simulink model "mat_double"  (R2020b)
settings: Solver=VariableStepAuto  StartTime=0.0  StopTime=10.0  RelTol=1e-3
values from neighbouring files (symbols this model uses):
  d1 = 0.5    [simu.m]    (also in simu_J1fix.m)
  d2 = 0.5    [simu.m]    (also in simu_J1fix.m)
  is_tm1 = 1    [simu.m]    (also in simu_J1fix.m)
  is_tm2 = 1    [simu.m]    (also in simu_J1fix.m)
  J1 = 1    [simu.m]    (also in simu_J1fix.m)
  J2 = 1    [simu.m]    (also in simu_J1fix.m = 0.8)
  k1 = 100    [simu.m]    (also in simu_J1fix.m)
  k2 = 100    [simu.m]    (also in simu_J1fix.m = 80)
undefined symbols (not defined in the file or in its folder): X, Y, Z
libraries: sm_lib x25, nesl_utility x17, fl_lib x6
settings Model: Creator=BearHsia  LastModifiedBy=BearHsia
settings ExplorerConfigSet: InternalSimMechanicsExplorerSettings="<ExplorerConfiguration><canonicalview>aerospace</canonicalview><AnimationSetting><BasePlaybackSpeed>1.0</BasePlaybackSpeed><PlaybackSpeedFactor>1.0</PlaybackSpeedFactor></AnimationSetting><TilePanel><TileInfo><Tiles Columns=\"1\" Count=\"1\" Rows=\"1\"><Column Weight=\"1\"/><Row Weight=\"1\"/><Tile Height=\"1\" Width=\"1\" X=\"0\" Y=\"0\"/></Tiles></TileInfo><SceneInfo><SceneViewer><BGColor><R>0.60000002384185791</R><G>0.60000002384185791</G><B>0.60000002384185791</B></BGColor><Camera><DoPerspective>off</DoPerspective><Position><X>0.0536048974703797823</X><Y>-0.0148520376451683166</Y><Z>1.01248960387817566</Z></Position><Center><X>0.0543519392340099453</X><Y>0.0174866883236047335</Y><Z>0.0130129164405163693</Z></Center><Up><X>-0.00285720568225904682</X><Y>0.999472955665096308</Y><Z>0.0323364696552736336</Z></Up><ViewLimDist>1</ViewLimDist><YLim>0.224098919359438681</YLim><XLim>0.18381667559028339</XLim></Camera></SceneViewer></SceneInfo></TilePanel><MechEditorPanel><Cameras/><GfxPanelCameraMap/><VideoCreator><PlaybackSpeedRatio>1.0</PlaybackSpeedRatio><FrameRate>30</FrameRate><VideoFormat>Motion JPEG AVI</VideoFormat><FrameSize>auto</FrameSize></VideoCreator></MechEditorPanel></ExplorerConfiguration>"

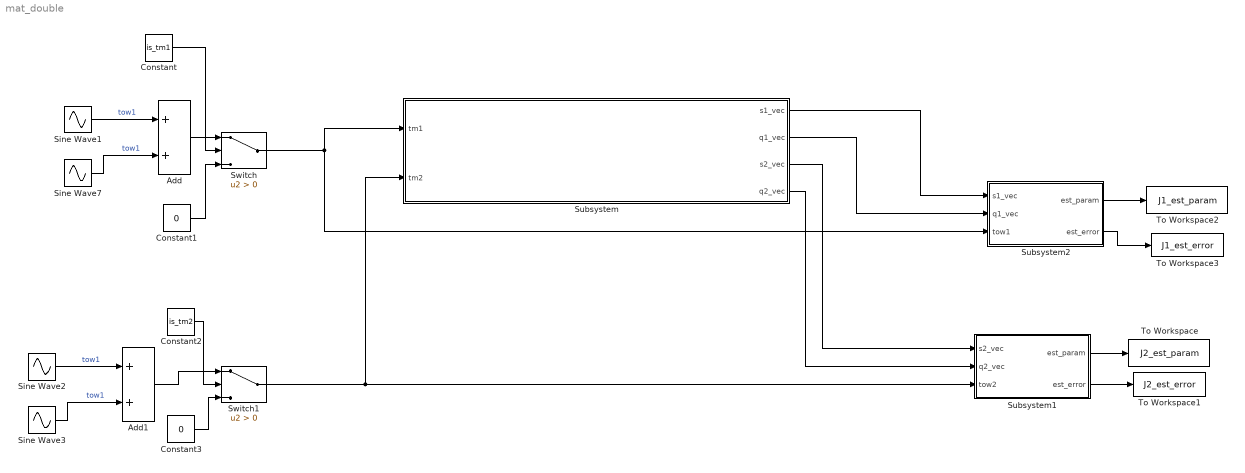
== system mat_double ==
  Add : Sum
  Add1 : Sum
  Constant : Constant  Value=is_tm1
  Constant1 : Constant  Value=0
  Constant2 : Constant  Value=is_tm2
  Constant3 : Constant  Value=0
  Sine Wave1 : Sin  Frequency=0.5  SampleTime=0
  Sine Wave2 : Sin  Amplitude=0.5  Frequency=0.5  SampleTime=0
  Sine Wave3 : Sin  Amplitude=0.25  Frequency=0.1  SampleTime=0
  Sine Wave7 : Sin  Amplitude=0.5  Frequency=0.1  SampleTime=0
  Subsystem : Subsystem
  Subsystem1 : Subsystem
  Subsystem2 : Subsystem
  Switch : Switch  Criteria=u2 > Threshold
  Switch1 : Switch  Criteria=u2 > Threshold
  To Workspace : ToWorkspace  VariableName=J2_est_param  SaveFormat=Timeseries  SampleTime=-1
  To Workspace1 : ToWorkspace  VariableName=J2_est_error  SaveFormat=Timeseries  SampleTime=-1
  To Workspace2 : ToWorkspace  VariableName=J1_est_param  SaveFormat=Timeseries  SampleTime=-1
  To Workspace3 : ToWorkspace  VariableName=J1_est_error  SaveFormat=Timeseries  SampleTime=-1
  wires:
  Constant1/1 -> Switch/3
  Constant/1 -> Switch/2
  Add/1 -> Switch/1
  Sine Wave7/1 -> Add/2  "tow1"
  Sine Wave1/1 -> Add/1  "tow1"
  Switch/1 -> Subsystem2/3(tow1), Subsystem/1(tm1)
  Subsystem2/2(est_error) -> To Workspace3/1
  Subsystem2/1(est_param) -> To Workspace2/1
  Subsystem/1(s1_vec) -> Subsystem2/1(s1_vec)
  Subsystem/2(q1_vec) -> Subsystem2/2(q1_vec)
  Add1/1 -> Switch1/1
  Constant2/1 -> Switch1/2
  Constant3/1 -> Switch1/3
  Sine Wave2/1 -> Add1/1  "tow1"
  Sine Wave3/1 -> Add1/2  "tow1"
  Switch1/1 -> Subsystem/2(tm2), Subsystem1/3(tow2)
  Subsystem1/1(est_param) -> To Workspace/1
  Subsystem1/2(est_error) -> To Workspace1/1
  Subsystem/3(s2_vec) -> Subsystem1/1(s2_vec)
  Subsystem/4(q2_vec) -> Subsystem1/2(q2_vec)

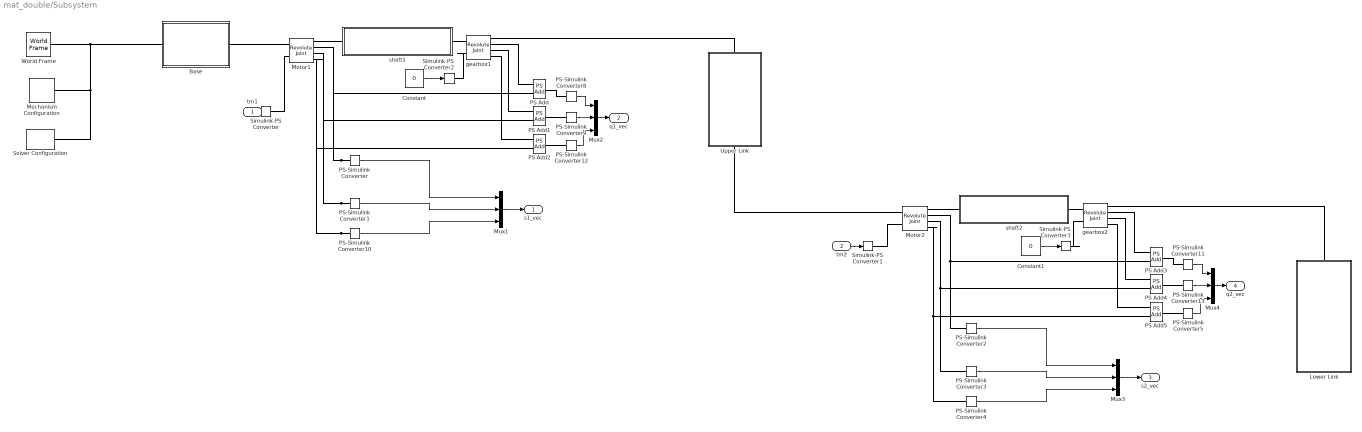
== system mat_double/Subsystem ==
  tm1 : Inport
  tm2 : Inport  Port=2
  Base : Subsystem  mask(Double Pendulum Base){R=6, T=0.5, rp=0.5, clr=[0.5 0.5 0.5], img_file=sm_dpen_base.png}
      mask prompts: R "Base radius (cm):"; T "Base thickness (cm):"; rp "Peg radius (cm):"; clr "Base color:"; img_file "Image file:"
      mask help: Base body of the double pendulum mechanism.
      mask Display: image(imread(img_file))
  Constant : Constant  Value=0
  Constant1 : Constant  Value=0
  Lower Link : Subsystem  mask(Lower Link){Ro=1200, L=20, W=2, T=0.5, r=0.5, clr=[1.0 0.2 0.2], img_file=sm_dpen_lower_link.png}
      mask prompts: Ro "Link density (kg/m^3):"; L "Link length (cm):"; W "Link width (cm):"; T "Link thickness (cm):"; r "Peg/Hole radius (cm):"; clr "Link color:"; img_file "Link image file:"
      mask help: Lower link of the pendulum mechanism.
      mask init:
      | % Main link cross-section
      | top_xsec = [L/2 W/2; -L/2 W/2];
      | theta = (90:-1:-90)*pi/180;
      | semi_hole_xsec = [-L/2+r*cos(theta') r*sin(theta')];
      | bottom_xsec = [-L/2 -W/2; L/2 -W/2];
      | theta = (-89:1:89)*pi/180;
      | right_end_xsec = [L/2+(W/2)*cos(theta') (W/2)*sin(theta')];
      | link_x_section = [ top_xsec; semi_hole_xsec; bottom_xsec; right_end_xsec];
      | 
      | % Left end cap cross-section
      | theta = (90:1:270)*pi/180;
      | outer_xsec = [(W/2)*cos(theta') (W/2)*sin(theta')];
      | theta = (270:-1:90)*pi/180;
      | inner_xsec = [r*cos(theta') r*sin(theta')];
      | left_end_x_section = [outer_xsec; inner_xsec];
      mask Display: image(imread(img_file));
  Mechanism Configuration : sm_lib/Utilities/Mechanism Configuration  UniformGravity=Constant  GravityVector=[0 -9.81 0]  GravityVectorUnits=m/s^2  GravityUnits=m/s^2  LinearizationDelta=0.001  JointModeTransitionNonlinearIterations=2
      settings: SourceProductName=Multibody
  Motor1 : sm_lib/Joints/Revolute Joint  JointMode=Normal  SenseConstraintForce=off  SenseConstraintForceX=off  SenseConstraintForceY=off  SenseConstraintForceZ=off  SenseConstraintTorque=off  SenseConstraintTorqueX=off  SenseConstraintTorqueY=off  SenseConstraintTorqueZ=off  SenseTotalForce=off  SenseTotalForceX=off  SenseTotalForceY=off  SenseTotalForceZ=off  SenseTotalTorque=off  SenseTotalTorqueX=off  SenseTotalTorqueY=off  SenseTotalTorqueZ=off  CompositeWrenchDir=FollowerOnBase  CompositeWrenchFrame=BaseFrame  EquilibriumPosition=0  EquilibriumPositionUnits=rad  SpringStiffness=0  SpringStiffnessUnits=N*m/rad  DampingCoefficient=0  DampingCoefficientUnits=N*m/(rad/s)  TorqueActuationMode=InputTorque  MotionActuationMode=ComputedMotion  SensePosition=on  SenseVelocity=on  SenseAcceleration=on  SenseTorqueForce=off  SenseLowerLimitTorqueForce=off  SenseUpperLimitTorqueForce=off  LowerLimitSpecify=off  LowerLimitBound=-90  LowerLimitBoundUnits=deg  LowerLimitStiffness=1e4  LowerLimitStiffnessUnits=N*m/deg  LowerLimitDamping=10  LowerLimitDampingUnits=N*m/(deg/s)  LowerLimitTransitionRegionWidth=0.1  LowerLimitTransitionRegionWidthUnits=deg  UpperLimitSpecify=off  UpperLimitBound=90  UpperLimitBoundUnits=deg  UpperLimitStiffness=1e4  UpperLimitStiffnessUnits=N*m/deg  UpperLimitDamping=10  UpperLimitDampingUnits=N*m/(deg/s)  UpperLimitTransitionRegionWidth=0.1  UpperLimitTransitionRegionWidthUnits=deg  PositionTargetSpecify=on  PositionTargetPriority=High  PositionTargetValue=0  PositionTargetValueUnits=rad  VelocityTargetSpecify=off  VelocityTargetPriority=High  VelocityTargetValue=0  VelocityTargetValueUnits=deg/s
  Motor2 : sm_lib/Joints/Revolute Joint  JointMode=Normal  SenseConstraintForce=off  SenseConstraintForceX=off  SenseConstraintForceY=off  SenseConstraintForceZ=off  SenseConstraintTorque=off  SenseConstraintTorqueX=off  SenseConstraintTorqueY=off  SenseConstraintTorqueZ=off  SenseTotalForce=off  SenseTotalForceX=off  SenseTotalForceY=off  SenseTotalForceZ=off  SenseTotalTorque=off  SenseTotalTorqueX=off  SenseTotalTorqueY=off  SenseTotalTorqueZ=off  CompositeWrenchDir=FollowerOnBase  CompositeWrenchFrame=BaseFrame  EquilibriumPosition=0  EquilibriumPositionUnits=rad  SpringStiffness=0  SpringStiffnessUnits=N*m/rad  DampingCoefficient=0  DampingCoefficientUnits=N*m/(rad/s)  TorqueActuationMode=InputTorque  MotionActuationMode=ComputedMotion  SensePosition=on  SenseVelocity=on  SenseAcceleration=on  SenseTorqueForce=off  SenseLowerLimitTorqueForce=off  SenseUpperLimitTorqueForce=off  LowerLimitSpecify=off  LowerLimitBound=-90  LowerLimitBoundUnits=deg  LowerLimitStiffness=1e4  LowerLimitStiffnessUnits=N*m/deg  LowerLimitDamping=10  LowerLimitDampingUnits=N*m/(deg/s)  LowerLimitTransitionRegionWidth=0.1  LowerLimitTransitionRegionWidthUnits=deg  UpperLimitSpecify=off  UpperLimitBound=90  UpperLimitBoundUnits=deg  UpperLimitStiffness=1e4  UpperLimitStiffnessUnits=N*m/deg  UpperLimitDamping=10  UpperLimitDampingUnits=N*m/(deg/s)  UpperLimitTransitionRegionWidth=0.1  UpperLimitTransitionRegionWidthUnits=deg  PositionTargetSpecify=on  PositionTargetPriority=High  PositionTargetValue=0  PositionTargetValueUnits=rad  VelocityTargetSpecify=off  VelocityTargetPriority=High  VelocityTargetValue=0  VelocityTargetValueUnits=deg/s
  Mux{1..4} (4 alike) : Mux  Inputs=3
  PS Add{,1..5} (6 alike) : fl_lib/Physical Signals/Functions/PS Add
  PS-Simulink Converter{,1..5,8..13} (12 alike) : nesl_utility/PS-Simulink Converter  PhysicalDomain=network_engine_domain  SubClassName=ps_output  LeftPortType=input  RightPortType=output  PseudoPeriodic=off  Frequencies=[]  Unit=inherit  AffineConversion=off
  Simulink-PS Converter{,1..3} (4 alike) : nesl_utility/Simulink-PS Converter  PhysicalDomain=network_engine_domain  SubClassName=ps_input  LeftPortType=input  RightPortType=output  PseudoPeriodic=off  Frequencies=[]  NoiseDistribution=none  NoiseParameters=[]  Unit=1  AffineConversion=off  FilteringAndDerivatives=provide  SimscapeFilterOrder=1  InputFilterTimeConstant=0.001  UdotUserProvided=0
  Solver Configuration : nesl_utility/Solver Configuration  PhysicalDomain=network_engine_domain  SubClassName=solver  LeftPortType=input  RightPortType=generic  Tones=[]  Harmonics=[]  SimulateNoise=off  Profile=off  UseLocalSampling=off  EnableSwitchedLinearOptims=on  FrequencyDomain=off  UseCCode=off  RelTol=0.001  AbsTol=1e-06  MinStep=1e-09  ToWorkspace=off  RevertToSquareIcSolve=off  NumHomotopyIterations=100  PhasorMode=off  PhasorModeNumHarmonics=1  DoDC=off  ResidualTolerance=1e-9  UseLocalSolver=off  LocalSolverChoice=NE_BACKWARD_EULER_ADVANCER  LocalSolverSampleTime=.001  DoFixedCost=off  MaxNonlinIter=3  MaxModeIter=2  ComputeImpulses=off  ImpulseIterations=2  LinearAlgebra=Sparse  EquationFormulation=NE_TIME_EF  DelaysMemoryBudget=1024  AutomaticFiltering=on  FilteringTimeConstant=0.001  PartitionStorageMethod=AS_NEEDED  PartitionMemoryBudget=1024  PartitionMethod=FAST
      settings: SourceProductName=Utilities
  Upper Link : Subsystem  mask(Upper Link){Ro=1000, L=14, W=2, T=0.5, r=0.5, clr=[0.0 0.6 0.8], img_file=sm_dpen_upper_link.png}
      mask prompts: Ro "Link density (kg/m^3):"; L "Link length (cm):"; W "Link width (cm):"; T "Link thickness (cm):"; r "Peg/Hole radius (cm):"; clr "Link color:"; img_file "Link image file:"
      mask help: Upper link of the double pendulum mechanism
      mask init: same as mat_double/Subsystem/Lower Link
      mask Display: image(imread(img_file));
  World Frame : sm_lib/Frames and Transforms/World Frame
      settings: SourceProductName=Multibody
  gearbox1 : sm_lib/Joints/Revolute Joint  JointMode=Normal  SenseConstraintForce=off  SenseConstraintForceX=off  SenseConstraintForceY=off  SenseConstraintForceZ=off  SenseConstraintTorque=off  SenseConstraintTorqueX=off  SenseConstraintTorqueY=off  SenseConstraintTorqueZ=off  SenseTotalForce=off  SenseTotalForceX=off  SenseTotalForceY=off  SenseTotalForceZ=off  SenseTotalTorque=off  SenseTotalTorqueX=off  SenseTotalTorqueY=off  SenseTotalTorqueZ=off  CompositeWrenchDir=FollowerOnBase  CompositeWrenchFrame=BaseFrame  EquilibriumPosition=0  EquilibriumPositionUnits=rad  SpringStiffness=k1  SpringStiffnessUnits=N*m/rad  DampingCoefficient=d1  DampingCoefficientUnits=N*m/(rad/s)  TorqueActuationMode=InputTorque  MotionActuationMode=ComputedMotion  SensePosition=on  SenseVelocity=on  SenseAcceleration=on  SenseTorqueForce=off  SenseLowerLimitTorqueForce=off  SenseUpperLimitTorqueForce=off  LowerLimitSpecify=off  LowerLimitBound=-90  LowerLimitBoundUnits=deg  LowerLimitStiffness=1e4  LowerLimitStiffnessUnits=N*m/deg  LowerLimitDamping=10  LowerLimitDampingUnits=N*m/(deg/s)  LowerLimitTransitionRegionWidth=0.1  LowerLimitTransitionRegionWidthUnits=deg  UpperLimitSpecify=off  UpperLimitBound=90  UpperLimitBoundUnits=deg  UpperLimitStiffness=1e4  UpperLimitStiffnessUnits=N*m/deg  UpperLimitDamping=10  UpperLimitDampingUnits=N*m/(deg/s)  UpperLimitTransitionRegionWidth=0.1  UpperLimitTransitionRegionWidthUnits=deg  PositionTargetSpecify=on  PositionTargetPriority=High  PositionTargetValue=0  PositionTargetValueUnits=rad  VelocityTargetSpecify=off  VelocityTargetPriority=High  VelocityTargetValue=0  VelocityTargetValueUnits=deg/s
  gearbox2 : sm_lib/Joints/Revolute Joint  JointMode=Normal  SenseConstraintForce=off  SenseConstraintForceX=off  SenseConstraintForceY=off  SenseConstraintForceZ=off  SenseConstraintTorque=off  SenseConstraintTorqueX=off  SenseConstraintTorqueY=off  SenseConstraintTorqueZ=off  SenseTotalForce=off  SenseTotalForceX=off  SenseTotalForceY=off  SenseTotalForceZ=off  SenseTotalTorque=off  SenseTotalTorqueX=off  SenseTotalTorqueY=off  SenseTotalTorqueZ=off  CompositeWrenchDir=FollowerOnBase  CompositeWrenchFrame=BaseFrame  EquilibriumPosition=0  EquilibriumPositionUnits=rad  SpringStiffness=k2  SpringStiffnessUnits=N*m/rad  DampingCoefficient=d2  DampingCoefficientUnits=N*m/(rad/s)  TorqueActuationMode=InputTorque  MotionActuationMode=ComputedMotion  SensePosition=on  SenseVelocity=on  SenseAcceleration=on  SenseTorqueForce=off  SenseLowerLimitTorqueForce=off  SenseUpperLimitTorqueForce=off  LowerLimitSpecify=off  LowerLimitBound=-90  LowerLimitBoundUnits=deg  LowerLimitStiffness=1e4  LowerLimitStiffnessUnits=N*m/deg  LowerLimitDamping=10  LowerLimitDampingUnits=N*m/(deg/s)  LowerLimitTransitionRegionWidth=0.1  LowerLimitTransitionRegionWidthUnits=deg  UpperLimitSpecify=off  UpperLimitBound=90  UpperLimitBoundUnits=deg  UpperLimitStiffness=1e4  UpperLimitStiffnessUnits=N*m/deg  UpperLimitDamping=10  UpperLimitDampingUnits=N*m/(deg/s)  UpperLimitTransitionRegionWidth=0.1  UpperLimitTransitionRegionWidthUnits=deg  PositionTargetSpecify=on  PositionTargetPriority=High  PositionTargetValue=0  PositionTargetValueUnits=rad  VelocityTargetSpecify=off  VelocityTargetPriority=High  VelocityTargetValue=0  VelocityTargetValueUnits=deg/s
  shaft1 : Subsystem  mask{rgb=[0 1 0], Ixx=0, Iyy=0, Izz=J1, M=0.1, L=0.2, W=0.004, H=0.004}
      mask prompts: rgb "Color [R G B]"
  shaft2 : Subsystem  mask{rgb=[0 1 0], Ixx=0, Iyy=0, Izz=J2, M=0.1, L=0.2, W=0.004, H=0.004}
      mask prompts: rgb "Color [R G B]"
  s1_vec : Outport
  q1_vec : Outport  Port=2
  s2_vec : Outport  Port=3
  q2_vec : Outport  Port=4
  wires:
  PS-Simulink Converter/1 -> Mux1/1
  PS-Simulink Converter8/1 -> Mux2/1
  PS-Simulink Converter9/1 -> Mux2/2
  Constant/1 -> Simulink-PS Converter2/1
  Mux2/1 -> q1_vec/1
  PS-Simulink Converter1/1 -> Mux1/2
  PS-Simulink Converter10/1 -> Mux1/3
  tm1/1 -> Simulink-PS Converter/1
  Mux1/1 -> s1_vec/1
  PS-Simulink Converter12/1 -> Mux2/3
  Constant1/1 -> Simulink-PS Converter3/1
  PS-Simulink Converter11/1 -> Mux4/1
  PS-Simulink Converter4/1 -> Mux3/3
  PS-Simulink Converter3/1 -> Mux3/2
  Mux3/1 -> s2_vec/1
  Mux4/1 -> q2_vec/1
  PS-Simulink Converter13/1 -> Mux4/2
  PS-Simulink Converter2/1 -> Mux3/1
  PS-Simulink Converter5/1 -> Mux4/3
  tm2/1 -> Simulink-PS Converter1/1
  connections:
  Base/RConn1 -- Motor1/LConn1
  Mechanism Configuration/RConn1 -- Solver Configuration/RConn1 -- Base/LConn1 -- World Frame/RConn1
  Motor2/LConn1 -- Upper Link/RConn1
  gearbox1/RConn1 -- Upper Link/LConn1
  PS-Simulink Converter/LConn1 -- Motor1/RConn2 -- PS Add/LConn2
  PS-Simulink Converter1/LConn1 -- Motor1/RConn3 -- PS Add1/LConn2
  PS-Simulink Converter10/LConn1 -- Motor1/RConn4 -- PS Add2/LConn2
  PS Add1/RConn1 -- PS-Simulink Converter9/LConn1
  shaft1/LConn1 -- Motor1/RConn1
  gearbox1/RConn2 -- PS Add/LConn1
  gearbox1/RConn4 -- PS Add2/LConn1
  Simulink-PS Converter/RConn1 -- Motor1/LConn2
  shaft1/RConn1 -- gearbox1/LConn1
  gearbox1/LConn2 -- Simulink-PS Converter2/RConn1
  PS Add/RConn1 -- PS-Simulink Converter8/LConn1
  gearbox1/RConn3 -- PS Add1/LConn1
  PS-Simulink Converter12/LConn1 -- PS Add2/RConn1
  PS Add4/LConn2 -- PS-Simulink Converter3/LConn1 -- Motor2/RConn3
  PS Add5/LConn2 -- PS-Simulink Converter4/LConn1 -- Motor2/RConn4
  PS Add3/LConn2 -- PS-Simulink Converter2/LConn1 -- Motor2/RConn2
  Simulink-PS Converter1/RConn1 -- Motor2/LConn2
  Simulink-PS Converter3/RConn1 -- gearbox2/LConn2
  shaft2/RConn1 -- gearbox2/LConn1
  shaft2/LConn1 -- Motor2/RConn1
  gearbox2/RConn4 -- PS Add5/LConn1
  gearbox2/RConn2 -- PS Add3/LConn1
  PS-Simulink Converter5/LConn1 -- PS Add5/RConn1
  gearbox2/RConn3 -- PS Add4/LConn1
  PS Add3/RConn1 -- PS-Simulink Converter11/LConn1
  Lower Link/LConn1 -- gearbox2/RConn1
  PS Add4/RConn1 -- PS-Simulink Converter13/LConn1

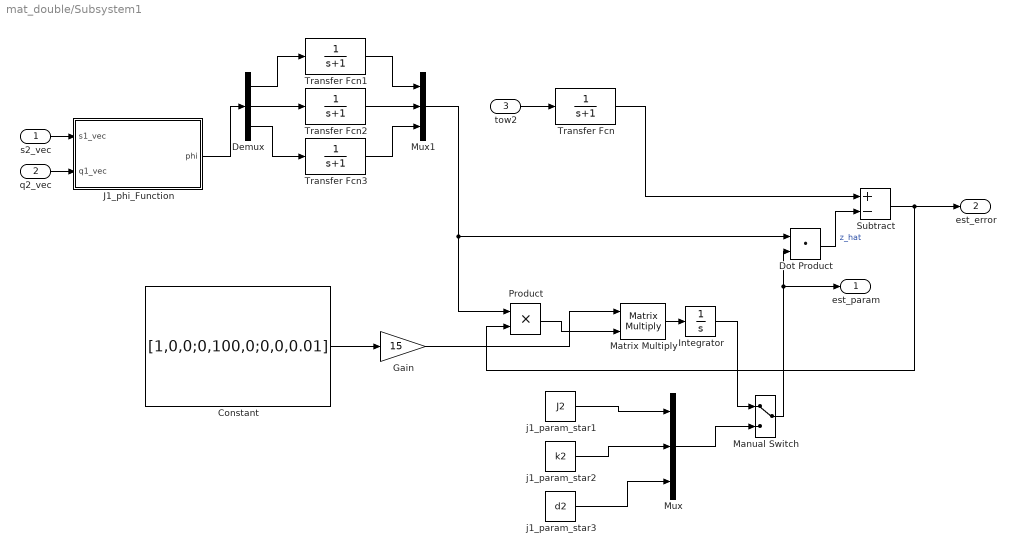
== system mat_double/Subsystem1 ==
  s2_vec : Inport
  q2_vec : Inport  Port=2
  tow2 : Inport  Port=3
  Constant : Constant  Value=[1,0,0;0,100,0;0,0,0.01]
  Demux : Demux  Outputs=3
  Dot Product : DotProduct  InputSameDT=on  OutDataTypeStr=Inherit: Inherit via internal rule
  Gain : Gain  Gain=15
  Integrator : Integrator  InitialCondition=[0.0001;0.0001;0.0001]
  J1_phi_Function : MATLAB Function  TreatAsAtomicUnit=on
  Manual Switch : ManualSwitch
  Matrix Multiply : Product  Multiplication=Matrix(*)
  Mux : Mux  Inputs=3
  Mux1 : Mux  Inputs=3
  Product : Product
  Subtract : Sum  Inputs=+-
  Transfer Fcn{,1..3} (4 alike) : TransferFcn  Denominator=[1 1]
  j1_param_star1 : Constant  Value=J2
  j1_param_star2 : Constant  Value=k2
  j1_param_star3 : Constant  Value=d2
  est_param : Outport
  est_error : Outport  Port=2
  wires:
  q2_vec/1 -> J1_phi_Function/2(q1_vec)
  s2_vec/1 -> J1_phi_Function/1(s1_vec)
  Integrator/1 -> Manual Switch/1
  tow2/1 -> Transfer Fcn/1
  Dot Product/1 -> Subtract/2  "z_hat"
  Matrix Multiply/1 -> Integrator/1
  Subtract/1 -> est_error/1, Product/2
  j1_param_star1/1 -> Mux/1
  j1_param_star2/1 -> Mux/2
  j1_param_star3/1 -> Mux/3
  Mux/1 -> Manual Switch/2
  Product/1 -> Matrix Multiply/2
  Constant/1 -> Gain/1
  Gain/1 -> Matrix Multiply/1
  J1_phi_Function/1(phi) -> Demux/1
  Manual Switch/1 -> est_param/1, Dot Product/2
  Transfer Fcn/1 -> Subtract/1
  Transfer Fcn1/1 -> Mux1/1
  Transfer Fcn2/1 -> Mux1/2
  Transfer Fcn3/1 -> Mux1/3
  Demux/3 -> Transfer Fcn3/1
  Demux/2 -> Transfer Fcn2/1
  Demux/1 -> Transfer Fcn1/1
  Mux1/1 -> Product/1, Dot Product/1

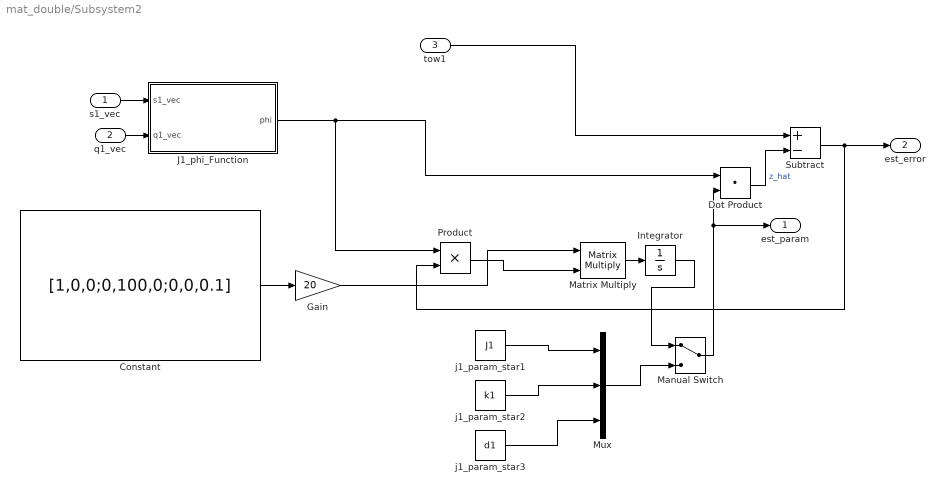
== system mat_double/Subsystem2 ==
  s1_vec : Inport
  q1_vec : Inport  Port=2
  tow1 : Inport  Port=3
  Constant : Constant  Value=[1,0,0;0,100,0;0,0,0.1]
  Dot Product : DotProduct  InputSameDT=on  OutDataTypeStr=Inherit: Inherit via internal rule
  Gain : Gain  Gain=20
  Integrator : Integrator  InitialCondition=[0;0;0]
  J1_phi_Function : MATLAB Function  TreatAsAtomicUnit=on
  Manual Switch : ManualSwitch
  Matrix Multiply : Product  Multiplication=Matrix(*)
  Mux : Mux  Inputs=3
  Product : Product
  Subtract : Sum  Inputs=+-
  j1_param_star1 : Constant  Value=J1
  j1_param_star2 : Constant  Value=k1
  j1_param_star3 : Constant  Value=d1
  est_param : Outport
  est_error : Outport  Port=2
  wires:
  q1_vec/1 -> J1_phi_Function/2(q1_vec)
  s1_vec/1 -> J1_phi_Function/1(s1_vec)
  Integrator/1 -> Manual Switch/1
  tow1/1 -> Subtract/1
  Dot Product/1 -> Subtract/2  "z_hat"
  Matrix Multiply/1 -> Integrator/1
  Subtract/1 -> est_error/1, Product/2
  j1_param_star1/1 -> Mux/1
  j1_param_star2/1 -> Mux/2
  j1_param_star3/1 -> Mux/3
  Mux/1 -> Manual Switch/2
  Product/1 -> Matrix Multiply/2
  Constant/1 -> Gain/1
  Gain/1 -> Matrix Multiply/1
  J1_phi_Function/1(phi) -> Dot Product/1, Product/1
  Manual Switch/1 -> est_param/1, Dot Product/2

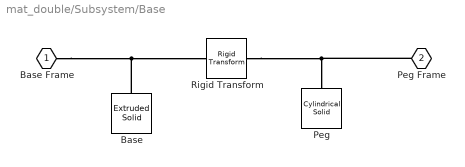
== system mat_double/Subsystem/Base ==
  Base : sm_lib/Body Elements/Extruded Solid  GraphicAmbientColor=[0.5 0.5 0.5]  BasedOnType=Density  CenterOfMass=[0 0 0]  CenterOfMassUnits=m  GraphicDiffuseColor=clr  ExportConvexHullGeometry=off  ExtrusionCrossSection=[1 1; -1 1; -1 -1; 1 -1]  ExtrusionCrossSectionUnits=m  Density=1  DensityUnits=kg/(m^3)  DoExposeReferenceFrame=on  GraphicEmissiveColor=[0.1 0.1 0.1]  ExportEntireGeometry=off  ExtrusionLength=T  ExtrusionLengthUnits=cm  ExtrusionType=Regular  SerializedFrames=<Frames/>  MarkerShape=Sphere  MarkerSize=1  GraphicType=FromGeometry  InertiaType=CalculateFromGeometry  Mass=1  MassUnits=kg  MomentsOfInertia=[1 1 1]  MomentsOfInertiaUnits=kg*m^2  PolygonNumSides=6  GraphicOpacity=1  PolygonOuterRadius=R  PolygonOuterRadiusUnits=cm  ProductsOfInertia=[0 0 0]  ProductsOfInertiaUnits=kg*m^2  GraphicShininess=24.0  GraphicSpecularColor=[0.2 0.2 0.2]  GraphicVisPropType=SimpleVisualProperties
      settings: SourceProductName=Multibody
  Peg : sm_lib/Body Elements/Cylindrical Solid  GraphicAmbientColor=[0.5 0.5 0.5]  BasedOnType=Density  CenterOfMass=[0 0 0]  CenterOfMassUnits=m  GraphicDiffuseColor=clr  CylinderLength=2*T  CylinderLengthUnits=cm  CylinderRadius=rp  CylinderRadiusUnits=cm  Density=1  DensityUnits=kg/(m^3)  DoExposeReferenceFrame=on  GraphicEmissiveColor=[0.1 0.1 0.1]  ExportEntireGeometry=off  SerializedFrames=<Frames/>  MarkerShape=Sphere  MarkerSize=1  GraphicType=FromGeometry  InertiaType=CalculateFromGeometry  Mass=1  MassUnits=kg  MomentsOfInertia=[1 1 1]  MomentsOfInertiaUnits=kg*m^2  GraphicOpacity=1  ProductsOfInertia=[0 0 0]  ProductsOfInertiaUnits=kg*m^2  GraphicShininess=24.0  GraphicSpecularColor=[0.2 0.2 0.2]  GraphicVisPropType=SimpleVisualProperties
      settings: SourceProductName=Multibody
  Rigid Transform : sm_lib/Frames and Transforms/Rigid Transform  TranslationMethod=StandardAxis  TranslationStandardOffset=3*T/2  TranslationLengthUnit=cm  TranslationStandardAxis=+Z  TranslationCartesianOffset=[0 0 0]  TranslationROffset=0  TranslationROffsetUnits=m  TranslationZOffset=0  TranslationZOffsetUnits=m  TranslationThetaOffset=0  TranslationThetaOffsetUnits=deg  RotationMethod=None  RotationAngleUnits=deg  RotationStandardAxis=+Z  RotationAngle=0  RotationArbitraryAxis=[0 0 1]  FollAlignAxisA=+X  BaseAlignAxisA=+Y  FollAlignAxisB=+Y  BaseAlignAxisB=+Z  RotationSequenceAxes=FollowerAxes  RotationSequence=XYX  RotationSequenceAngles=[0 0 0]  RotationSequenceAnglesUnits=deg  RotationMatrix=[1 0 0; 0 1 0; 0 0 1]
      settings: SourceProductName=Multibody
  Base Frame : PMIOPort  Side=Left
  Peg Frame : PMIOPort  Port=2  Side=Right
  connections:
  Base Frame/RConn1 -- Base/RConn1 -- Rigid Transform/LConn1
  Peg Frame/RConn1 -- Rigid Transform/RConn1 -- Peg/RConn1

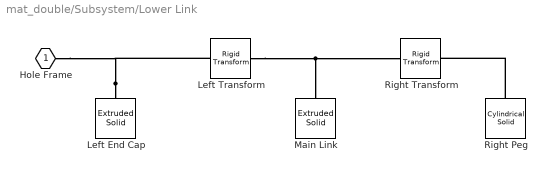
== system mat_double/Subsystem/Lower Link ==
  Left Transform : sm_lib/Frames and Transforms/Rigid Transform  TranslationMethod=StandardAxis  TranslationStandardOffset=L/2  TranslationLengthUnit=cm  TranslationStandardAxis=-X  TranslationCartesianOffset=[0 0 0]  TranslationROffset=0  TranslationROffsetUnits=m  TranslationZOffset=0  TranslationZOffsetUnits=m  TranslationThetaOffset=0  TranslationThetaOffsetUnits=deg  RotationMethod=None  RotationAngleUnits=deg  RotationStandardAxis=+Z  RotationAngle=0  RotationArbitraryAxis=[0 0 1]  FollAlignAxisA=+X  BaseAlignAxisA=+Y  FollAlignAxisB=+Y  BaseAlignAxisB=+Z  RotationSequenceAxes=FollowerAxes  RotationSequence=XYX  RotationSequenceAngles=[0 0 0]  RotationSequenceAnglesUnits=deg  RotationMatrix=[1 0 0; 0 1 0; 0 0 1]
      settings: SourceProductName=Multibody
  Left End Cap : sm_lib/Body Elements/Extruded Solid  GraphicAmbientColor=[0.5 0.5 0.5]  BasedOnType=Density  CenterOfMass=[0 0 0]  CenterOfMassUnits=m  GraphicDiffuseColor=clr  ExportConvexHullGeometry=off  ExtrusionCrossSection=left_end_x_section  ExtrusionCrossSectionUnits=cm  Density=Ro  DensityUnits=kg/m^3  DoExposeReferenceFrame=on  GraphicEmissiveColor=[0.1 0.1 0.1]  ExportEntireGeometry=off  ExtrusionLength=T  ExtrusionLengthUnits=cm  ExtrusionType=General  SerializedFrames=<Frames/>  MarkerShape=Sphere  MarkerSize=1  GraphicType=FromGeometry  InertiaType=CalculateFromGeometry  Mass=1  MassUnits=kg  MomentsOfInertia=[1 1 1]  MomentsOfInertiaUnits=kg*m^2  PolygonNumSides=1  GraphicOpacity=1  PolygonOuterRadius=1  PolygonOuterRadiusUnits=m  ProductsOfInertia=[0 0 0]  ProductsOfInertiaUnits=kg*m^2  GraphicShininess=24.0  GraphicSpecularColor=[0.2 0.2 0.2]  GraphicVisPropType=SimpleVisualProperties
      settings: SourceProductName=Multibody
  Main Link : sm_lib/Body Elements/Extruded Solid  GraphicAmbientColor=[0.5 0.5 0.5]  BasedOnType=Density  CenterOfMass=[0 0 0]  CenterOfMassUnits=m  GraphicDiffuseColor=clr  ExportConvexHullGeometry=off  ExtrusionCrossSection=link_x_section  ExtrusionCrossSectionUnits=cm  Density=Ro  DensityUnits=kg/m^3  DoExposeReferenceFrame=on  GraphicEmissiveColor=[0.1 0.1 0.1]  ExportEntireGeometry=off  ExtrusionLength=T  ExtrusionLengthUnits=cm  ExtrusionType=General  SerializedFrames=<Frames/>  MarkerShape=Sphere  MarkerSize=1  GraphicType=FromGeometry  InertiaType=CalculateFromGeometry  Mass=1  MassUnits=kg  MomentsOfInertia=[1 1 1]  MomentsOfInertiaUnits=kg*m^2  PolygonNumSides=1  GraphicOpacity=1  PolygonOuterRadius=1  PolygonOuterRadiusUnits=m  ProductsOfInertia=[0 0 0]  ProductsOfInertiaUnits=kg*m^2  GraphicShininess=24.0  GraphicSpecularColor=[0.2 0.2 0.2]  GraphicVisPropType=SimpleVisualProperties
      settings: SourceProductName=Multibody
  Right Peg : sm_lib/Body Elements/Cylindrical Solid  GraphicAmbientColor=[0.5 0.5 0.5]  BasedOnType=Density  CenterOfMass=[0 0 0]  CenterOfMassUnits=m  GraphicDiffuseColor=clr  CylinderLength=2*T  CylinderLengthUnits=cm  CylinderRadius=r  CylinderRadiusUnits=cm  Density=Ro  DensityUnits=kg/m^3  DoExposeReferenceFrame=on  GraphicEmissiveColor=[0.1 0.1 0.1]  ExportEntireGeometry=off  SerializedFrames=<Frames/>  MarkerShape=Sphere  MarkerSize=1  GraphicType=FromGeometry  InertiaType=CalculateFromGeometry  Mass=1  MassUnits=kg  MomentsOfInertia=[1 1 1]  MomentsOfInertiaUnits=kg*m^2  GraphicOpacity=1  ProductsOfInertia=[0 0 0]  ProductsOfInertiaUnits=kg*m^2  GraphicShininess=24.0  GraphicSpecularColor=[0.2 0.2 0.2]  GraphicVisPropType=SimpleVisualProperties
      settings: SourceProductName=Multibody
  Right Transform : sm_lib/Frames and Transforms/Rigid Transform  TranslationMethod=Cartesian  TranslationStandardOffset=0  TranslationLengthUnit=cm  TranslationStandardAxis=+Z  TranslationCartesianOffset=[L/2 0 3*T/2]  TranslationROffset=0  TranslationROffsetUnits=m  TranslationZOffset=0  TranslationZOffsetUnits=m  TranslationThetaOffset=0  TranslationThetaOffsetUnits=deg  RotationMethod=None  RotationAngleUnits=deg  RotationStandardAxis=+Z  RotationAngle=0  RotationArbitraryAxis=[0 0 1]  FollAlignAxisA=+X  BaseAlignAxisA=+Y  FollAlignAxisB=+Y  BaseAlignAxisB=+Z  RotationSequenceAxes=FollowerAxes  RotationSequence=XYX  RotationSequenceAngles=[0 0 0]  RotationSequenceAnglesUnits=deg  RotationMatrix=[1 0 0; 0 1 0; 0 0 1]
      settings: SourceProductName=Multibody
  Hole Frame : PMIOPort  Side=Left
  connections:
  Right Peg/RConn1 -- Right Transform/RConn1
  Left End Cap/RConn1 -- Hole Frame/RConn1 -- Left Transform/RConn1
  Left Transform/LConn1 -- Right Transform/LConn1 -- Main Link/RConn1

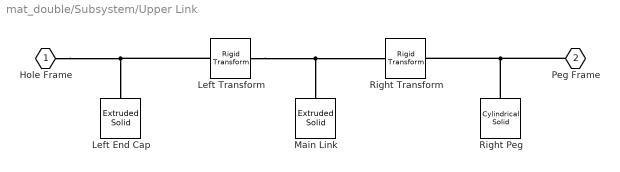
== system mat_double/Subsystem/Upper Link ==
  Left Transform : sm_lib/Frames and Transforms/Rigid Transform  TranslationMethod=StandardAxis  TranslationStandardOffset=L/2  TranslationLengthUnit=cm  TranslationStandardAxis=-X  TranslationCartesianOffset=[0 0 0]  TranslationROffset=0  TranslationROffsetUnits=m  TranslationZOffset=0  TranslationZOffsetUnits=m  TranslationThetaOffset=0  TranslationThetaOffsetUnits=deg  RotationMethod=None  RotationAngleUnits=deg  RotationStandardAxis=+Z  RotationAngle=0  RotationArbitraryAxis=[0 0 1]  FollAlignAxisA=+X  BaseAlignAxisA=+Y  FollAlignAxisB=+Y  BaseAlignAxisB=+Z  RotationSequenceAxes=FollowerAxes  RotationSequence=XYX  RotationSequenceAngles=[0 0 0]  RotationSequenceAnglesUnits=deg  RotationMatrix=[1 0 0; 0 1 0; 0 0 1]
      settings: SourceProductName=Multibody
  Left End Cap : sm_lib/Body Elements/Extruded Solid  GraphicAmbientColor=[0.5 0.5 0.5]  BasedOnType=Density  CenterOfMass=[0 0 0]  CenterOfMassUnits=m  GraphicDiffuseColor=clr  ExportConvexHullGeometry=off  ExtrusionCrossSection=left_end_x_section  ExtrusionCrossSectionUnits=cm  Density=Ro  DensityUnits=kg/m^3  DoExposeReferenceFrame=on  GraphicEmissiveColor=[0.1 0.1 0.1]  ExportEntireGeometry=off  ExtrusionLength=T  ExtrusionLengthUnits=cm  ExtrusionType=General  SerializedFrames=<Frames/>  MarkerShape=Sphere  MarkerSize=1  GraphicType=FromGeometry  InertiaType=CalculateFromGeometry  Mass=1  MassUnits=kg  MomentsOfInertia=[1 1 1]  MomentsOfInertiaUnits=kg*m^2  PolygonNumSides=1  GraphicOpacity=1  PolygonOuterRadius=1  PolygonOuterRadiusUnits=m  ProductsOfInertia=[0 0 0]  ProductsOfInertiaUnits=kg*m^2  GraphicShininess=24.0  GraphicSpecularColor=[0.2 0.2 0.2]  GraphicVisPropType=SimpleVisualProperties
      settings: SourceProductName=Multibody
  Main Link : sm_lib/Body Elements/Extruded Solid  GraphicAmbientColor=[0.5 0.5 0.5]  BasedOnType=Density  CenterOfMass=[0 0 0]  CenterOfMassUnits=m  GraphicDiffuseColor=clr  ExportConvexHullGeometry=off  ExtrusionCrossSection=link_x_section  ExtrusionCrossSectionUnits=cm  Density=Ro  DensityUnits=kg/m^3  DoExposeReferenceFrame=on  GraphicEmissiveColor=[0.1 0.1 0.1]  ExportEntireGeometry=off  ExtrusionLength=T  ExtrusionLengthUnits=cm  ExtrusionType=General  SerializedFrames=<Frames/>  MarkerShape=Sphere  MarkerSize=1  GraphicType=FromGeometry  InertiaType=CalculateFromGeometry  Mass=1  MassUnits=kg  MomentsOfInertia=[1 1 1]  MomentsOfInertiaUnits=kg*m^2  PolygonNumSides=1  GraphicOpacity=1  PolygonOuterRadius=1  PolygonOuterRadiusUnits=m  ProductsOfInertia=[0 0 0]  ProductsOfInertiaUnits=kg*m^2  GraphicShininess=24.0  GraphicSpecularColor=[0.2 0.2 0.2]  GraphicVisPropType=SimpleVisualProperties
      settings: SourceProductName=Multibody
  Right Peg : sm_lib/Body Elements/Cylindrical Solid  GraphicAmbientColor=[0.5 0.5 0.5]  BasedOnType=Density  CenterOfMass=[0 0 0]  CenterOfMassUnits=m  GraphicDiffuseColor=clr  CylinderLength=2*T  CylinderLengthUnits=cm  CylinderRadius=r  CylinderRadiusUnits=cm  Density=Ro  DensityUnits=kg/m^3  DoExposeReferenceFrame=on  GraphicEmissiveColor=[0.1 0.1 0.1]  ExportEntireGeometry=off  SerializedFrames=<Frames/>  MarkerShape=Sphere  MarkerSize=1  GraphicType=FromGeometry  InertiaType=CalculateFromGeometry  Mass=1  MassUnits=kg  MomentsOfInertia=[1 1 1]  MomentsOfInertiaUnits=kg*m^2  GraphicOpacity=1  ProductsOfInertia=[0 0 0]  ProductsOfInertiaUnits=kg*m^2  GraphicShininess=24.0  GraphicSpecularColor=[0.2 0.2 0.2]  GraphicVisPropType=SimpleVisualProperties
      settings: SourceProductName=Multibody
  Right Transform : sm_lib/Frames and Transforms/Rigid Transform  TranslationMethod=Cartesian  TranslationStandardOffset=0  TranslationLengthUnit=cm  TranslationStandardAxis=+Z  TranslationCartesianOffset=[L/2 0 3*T/2]  TranslationROffset=0  TranslationROffsetUnits=m  TranslationZOffset=0  TranslationZOffsetUnits=m  TranslationThetaOffset=0  TranslationThetaOffsetUnits=deg  RotationMethod=None  RotationAngleUnits=deg  RotationStandardAxis=+Z  RotationAngle=0  RotationArbitraryAxis=[0 0 1]  FollAlignAxisA=+X  BaseAlignAxisA=+Y  FollAlignAxisB=+Y  BaseAlignAxisB=+Z  RotationSequenceAxes=FollowerAxes  RotationSequence=XYX  RotationSequenceAngles=[0 0 0]  RotationSequenceAnglesUnits=deg  RotationMatrix=[1 0 0; 0 1 0; 0 0 1]
      settings: SourceProductName=Multibody
  Hole Frame : PMIOPort  Side=Left
  Peg Frame : PMIOPort  Port=2  Side=Right
  connections:
  Left Transform/LConn1 -- Right Transform/LConn1 -- Main Link/RConn1
  Hole Frame/RConn1 -- Left Transform/RConn1 -- Left End Cap/RConn1
  Peg Frame/RConn1 -- Right Peg/RConn1 -- Right Transform/RConn1

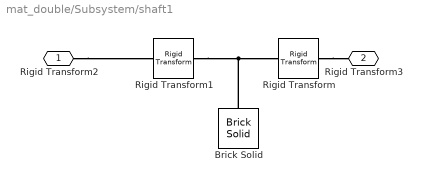
== system mat_double/Subsystem/shaft1 ==
  Brick Solid : sm_lib/Body Elements/Brick Solid  GraphicAmbientColor=[0.15 0.15 0.15 1.0]  BasedOnType=Density  BrickDimensions=[L W H]  BrickDimensionUnits=m  CenterOfMass=[0 0 0]  CenterOfMassUnits=m  GraphicDiffuseColor=rgb  Density=2700  DensityUnits=kg/m^3  DoExposeReferenceFrame=on  GraphicEmissiveColor=[0.0 0.0 0.0 1.0]  ExportEntireGeometry=off  SerializedFrames=<Frames/>  MarkerShape=Sphere  MarkerSize=10  GraphicType=FromGeometry  InertiaType=Custom  Mass=M  MassUnits=kg  MomentsOfInertia=[Ixx Iyy Izz]  MomentsOfInertiaUnits=kg*m^2  GraphicOpacity=1.0  ProductsOfInertia=[0 0 0]  ProductsOfInertiaUnits=kg*m^2  GraphicShininess=75  GraphicSpecularColor=[0.5 0.5 0.5 1.0]  GraphicVisPropType=SimpleVisualProperties
  Rigid Transform : sm_lib/Frames and Transforms/Rigid Transform  TranslationMethod=None  TranslationStandardOffset=0  TranslationLengthUnit=m  TranslationStandardAxis=+X  TranslationCartesianOffset=[0 0 0]  TranslationROffset=0  TranslationROffsetUnits=m  TranslationZOffset=0  TranslationZOffsetUnits=m  TranslationThetaOffset=0  TranslationThetaOffsetUnits=deg  RotationMethod=None  RotationAngleUnits=deg  RotationStandardAxis=+Z  RotationAngle=0.0  RotationArbitraryAxis=[0 0 1]  FollAlignAxisA=+X  BaseAlignAxisA=+Y  FollAlignAxisB=+Y  BaseAlignAxisB=+Z  RotationSequenceAxes=FollowerAxes  RotationSequence=XYX  RotationSequenceAngles=[0 0 0]  RotationSequenceAnglesUnits=deg  RotationMatrix=[1 0 0; 0 1 0; 0 0 1]
  Rigid Transform1 : sm_lib/Frames and Transforms/Rigid Transform  TranslationMethod=None  TranslationStandardOffset=0  TranslationLengthUnit=m  TranslationStandardAxis=-X  TranslationCartesianOffset=[0 0 0]  TranslationROffset=0  TranslationROffsetUnits=m  TranslationZOffset=0  TranslationZOffsetUnits=m  TranslationThetaOffset=0  TranslationThetaOffsetUnits=deg  RotationMethod=None  RotationAngleUnits=deg  RotationStandardAxis=-X  RotationAngle=0.0  RotationArbitraryAxis=[0 0 1]  FollAlignAxisA=+X  BaseAlignAxisA=+Y  FollAlignAxisB=+Y  BaseAlignAxisB=+Z  RotationSequenceAxes=FollowerAxes  RotationSequence=XYX  RotationSequenceAngles=[0 0 0]  RotationSequenceAnglesUnits=deg  RotationMatrix=[1 0 0; 0 1 0; 0 0 1]
  Rigid Transform2 : PMIOPort  Side=Left
  Rigid Transform3 : PMIOPort  Port=2  Side=Right
  connections:
  Rigid Transform1/LConn1 -- Rigid Transform/LConn1 -- Brick Solid/RConn1
  Rigid Transform/RConn1 -- Rigid Transform3/RConn1
  Rigid Transform2/RConn1 -- Rigid Transform1/RConn1

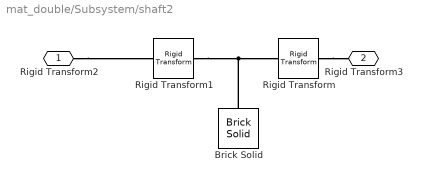
== system mat_double/Subsystem/shaft2 ==
  Brick Solid : sm_lib/Body Elements/Brick Solid  GraphicAmbientColor=[0.15 0.15 0.15 1.0]  BasedOnType=Density  BrickDimensions=[L W H]  BrickDimensionUnits=m  CenterOfMass=[0 0 0]  CenterOfMassUnits=m  GraphicDiffuseColor=rgb  Density=2700  DensityUnits=kg/m^3  DoExposeReferenceFrame=on  GraphicEmissiveColor=[0.0 0.0 0.0 1.0]  ExportEntireGeometry=off  SerializedFrames=<Frames/>  MarkerShape=Sphere  MarkerSize=10  GraphicType=FromGeometry  InertiaType=Custom  Mass=M  MassUnits=kg  MomentsOfInertia=[Ixx Iyy Izz]  MomentsOfInertiaUnits=kg*m^2  GraphicOpacity=1.0  ProductsOfInertia=[0 0 0]  ProductsOfInertiaUnits=kg*m^2  GraphicShininess=75  GraphicSpecularColor=[0.5 0.5 0.5 1.0]  GraphicVisPropType=SimpleVisualProperties
  Rigid Transform : sm_lib/Frames and Transforms/Rigid Transform  TranslationMethod=None  TranslationStandardOffset=0  TranslationLengthUnit=m  TranslationStandardAxis=+X  TranslationCartesianOffset=[0 0 0]  TranslationROffset=0  TranslationROffsetUnits=m  TranslationZOffset=0  TranslationZOffsetUnits=m  TranslationThetaOffset=0  TranslationThetaOffsetUnits=deg  RotationMethod=None  RotationAngleUnits=deg  RotationStandardAxis=+Z  RotationAngle=0.0  RotationArbitraryAxis=[0 0 1]  FollAlignAxisA=+X  BaseAlignAxisA=+Y  FollAlignAxisB=+Y  BaseAlignAxisB=+Z  RotationSequenceAxes=FollowerAxes  RotationSequence=XYX  RotationSequenceAngles=[0 0 0]  RotationSequenceAnglesUnits=deg  RotationMatrix=[1 0 0; 0 1 0; 0 0 1]
  Rigid Transform1 : sm_lib/Frames and Transforms/Rigid Transform  TranslationMethod=None  TranslationStandardOffset=0  TranslationLengthUnit=m  TranslationStandardAxis=-X  TranslationCartesianOffset=[0 0 0]  TranslationROffset=0  TranslationROffsetUnits=m  TranslationZOffset=0  TranslationZOffsetUnits=m  TranslationThetaOffset=0  TranslationThetaOffsetUnits=deg  RotationMethod=None  RotationAngleUnits=deg  RotationStandardAxis=-X  RotationAngle=0.0  RotationArbitraryAxis=[0 0 1]  FollAlignAxisA=+X  BaseAlignAxisA=+Y  FollAlignAxisB=+Y  BaseAlignAxisB=+Z  RotationSequenceAxes=FollowerAxes  RotationSequence=XYX  RotationSequenceAngles=[0 0 0]  RotationSequenceAnglesUnits=deg  RotationMatrix=[1 0 0; 0 1 0; 0 0 1]
  Rigid Transform2 : PMIOPort  Side=Left
  Rigid Transform3 : PMIOPort  Port=2  Side=Right
  connections:
  Rigid Transform1/LConn1 -- Rigid Transform/LConn1 -- Brick Solid/RConn1
  Rigid Transform/RConn1 -- Rigid Transform3/RConn1
  Rigid Transform2/RConn1 -- Rigid Transform1/RConn1

== matlab function mat_double/Subsystem1/J1_phi_Function ==
  data: s1_vec input; phi output; q1_vec input
function phi = J2_phi(s1_vec,q1_vec)
s1 = s1_vec(1);
s1_d = s1_vec(2);
s1_dd = s1_vec(3);
q1 = q1_vec(1);
q1_d = q1_vec(2);
q1_dd = q1_vec(3);

phi1 = s1_dd;
phi2 = s1-q1;
phi3 = s1_d-q1_d;

phi = [phi1;phi2;phi3];

== matlab function mat_double/Subsystem2/J1_phi_Function ==
  data: s1_vec input; phi output; q1_vec input
function phi = J1_phi(s1_vec,q1_vec)
s1 = s1_vec(1);
s1_d = s1_vec(2);
s1_dd = s1_vec(3);
q1 = q1_vec(1);
q1_d = q1_vec(2);
q1_dd = q1_vec(3);

phi1 = s1_dd;
phi2 = s1-q1;
phi3 = s1_d-q1_d;

phi = [phi1;phi2;phi3];
